simulink model "untitled"  (Simulink 7.6)
settings: Solver=VariableStepDiscrete  StartTime=0.0  StopTime=1000  RelTol=1e-3
values from neighbouring files (symbols this model uses):
  r = - obj.PENALTY    [TaskCompareWindWithSimulink.m]    (also in TaskCompareWindWithSimulinkW2D30.m)
undefined symbols (not defined in the file or in its folder): F, MIL, Moderate
libraries: aerolibwind2 x1, aerolibtransform2 x1
settings Model: Creator=rdenardi  LastModifiedBy=rdenardi

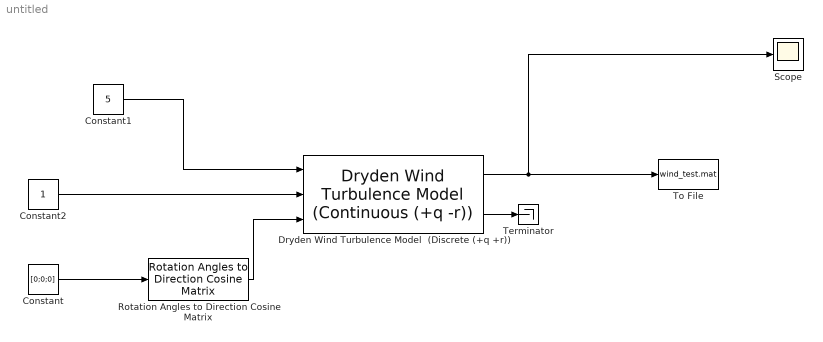
== system untitled ==
  Constant : Constant  Value=[0;0;0]  VectorParams1D=off
  Constant1 : Constant  Value=5
  Constant2 : Constant
  Dryden Wind Turbulence Model  (Discrete (+q +r)) : aerolibwind2/Dryden Wind Turbulence Model  (Continuous (+q -r))  SystemSampleTime=-1  units=English (Velocity in ft/s)  spec=MIL-F-8785C  model=Discrete Dryden (+q +r)  W20=1  Wdeg=0  TurbProb=10^-3 - Moderate  L_high=1000  Wingspan=0.5  ts=0.01  Seed=[23341 23342 23343 23344]  T_on=on
  Rotation Angles to Direction Cosine Matrix : aerolibtransform2/Rotation Angles to Direction Cosine Matrix  SystemSampleTime=-1  rotationOrder=ZYX
  Scope : Scope
  Terminator : Terminator
  To File : ToFile  Filename=wind_test.mat
  wires:
  Dryden Wind Turbulence Model  (Discrete (+q +r))/1 -> Scope/1, To File/1
  Dryden Wind Turbulence Model  (Discrete (+q +r))/2 -> Terminator/1
  Rotation Angles to Direction Cosine Matrix/1 -> Dryden Wind Turbulence Model  (Discrete (+q +r))/3
  Constant/1 -> Rotation Angles to Direction Cosine Matrix/1
  Constant1/1 -> Dryden Wind Turbulence Model  (Discrete (+q +r))/1
  Constant2/1 -> Dryden Wind Turbulence Model  (Discrete (+q +r))/2
